simulink model "sampleModel2073"  (R2023a)
settings: Solver=VariableStepAuto  StartTime=0.0  StopTime=10.0  RelTol=1e-3
libraries: hdlsllib x4, simulink x3
settings Model: Creator=user1  LastModifiedBy=user1

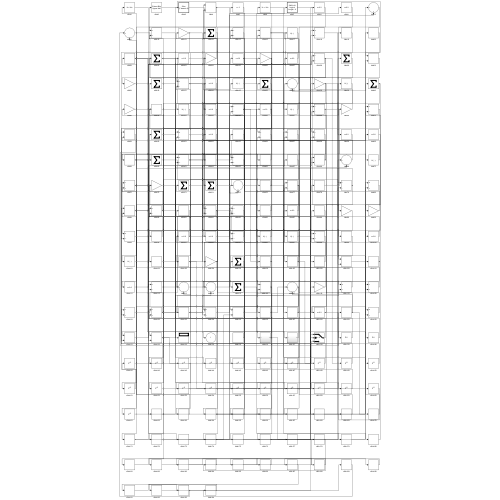
[thumbnail: Simulink's stored preview of the top-level diagram]
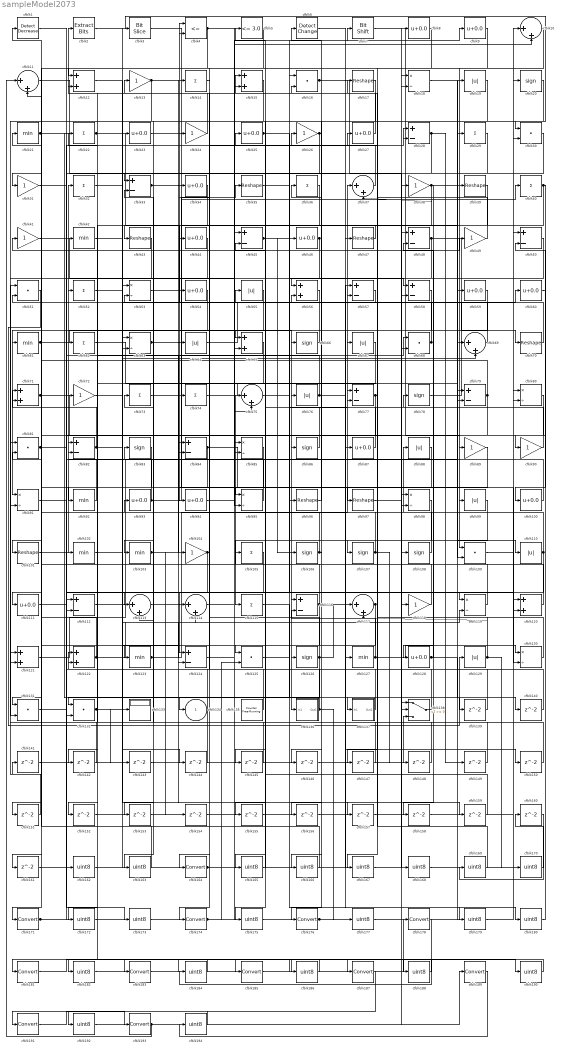
== system sampleModel2073 ==
  cfblk1 : simulink/Logic and Bit Operations/Detect Decrease  vinit=0.0  OutDataTypeStr=boolean
      settings: LibrarySourceBlock=|
      | hdlsllib/Logic and Bit
      | Operations/Detect
      | Decrease
  cfblk{10..11,37,69,75,113..114,117} (8 alike) : Sum  Inputs=|++
  cfblk{8..9,23,25,27,34,44,46,54,59..60,87,93..94,100,111,128} (17 alike) : Bias  Bias=0.0  SaturateOnIntegerOverflow=off
  cfblk{17,35,39,43,47,70,96..97,101} (9 alike) : Reshape
  cfblk{21,42,61,92,102..103,123,127} (8 alike) : MinMax
  cfblk{13,24,26,31,38,41,49,72,89..90,104,118} (12 alike) : Gain
  cfblk{14,22,29,32,36,40,52,62,73..74,105,115} (12 alike) : Sum  Inputs=+
  cfblk{20,66,78,83,86,106..108,126} (9 alike) : Signum
  cfblk{16,30,51,68,81,109,125,131..132} (9 alike) : DotProduct  OutDataTypeStr=Inherit: Inherit via internal rule
  cfblk{19,55,64,67,76,88,99,110,129} (9 alike) : Abs  SaturateOnIntegerOverflow=off
  cfblk{28,33,45,48,50,57..58,77,79,82,84,112,116,124} (14 alike) : Sum  Inputs=+-
  cfblk{18,53,63,80,85,91,95,98,119,130} (10 alike) : Product  Inputs=*/  RndMeth=Zero  SaturateOnIntegerOverflow=on
  cfblk{12,15,56,65,71,120..122} (8 alike) : Sum
  cfblk133 : Display
  cfblk135 : hdlsllib/Sources/Counter Free-Running  NumBits=16  tsamp=-1
  cfblk136 : Subsystem
      settings: LibrarySourceBlock=|
      | hdlsllib/Ports &
      | Subsystems/Subsystem
  cfblk137 : Subsystem
      settings: LibrarySourceBlock=|
      | hdlsllib/Ports &
      | Subsystems/Subsystem
  cfblk138 : Switch  SaturateOnIntegerOverflow=off  InputSameDT=off
  cfblk{139..161} (23 alike) : Delay  SampleTime=1
  cfblk{162..163,165..170,172..173,175,177,179..180,182,184,186,188,190,192,194} (21 alike) : DataTypeConversion  OutDataTypeStr=uint8  SaturateOnIntegerOverflow=off  RndMeth=Floor
  cfblk{164,171,174,176,178,181,183,185,187,189,191,193} (12 alike) : DataTypeConversion  SaturateOnIntegerOverflow=off  RndMeth=Floor
  cfblk2 : simulink/Logic and Bit Operations/Extract Bits  bitsToExtract=Upper half  numBits=8  bitIdxRange=[0 7]  outScalingMode=Preserve fixed-point scaling
      settings: LibrarySourceBlock=|
      | hdlsllib/Logic and Bit
      | Operations/Extract Bits
  cfblk3 : hdlsllib/Logic and Bit Operations/Bit Slice  lidx=7  ridx=0
  cfblk4 : RelationalOperator  Operator=<=  OutDataTypeStr=boolean  InputSameDT=off
  cfblk5 : hdlsllib/Logic and Bit Operations/Compare To Constant  relop=<=  const=3.0  OutDataTypeStr=boolean
  cfblk6 : simulink/Logic and Bit Operations/Detect Change  vinit=0  OutDataTypeStr=boolean
      settings: LibrarySourceBlock=|
      | hdlsllib/Logic and Bit
      | Operations/Detect
      | Change
  cfblk7 : hdlsllib/Logic and Bit Operations/Bit Shift  mode=Shift Left Logical  N=0
  cfblk134 : Outport  VectorParamsAs1DForOutWhenUnconnected=off
  wires:
  cfblk128/1 -> cfblk48/2, cfblk140/1
  cfblk21/1 -> cfblk137/1(In1), cfblk47/1, cfblk84/1
  cfblk93/1 -> cfblk55/1, cfblk12/2
  cfblk111/1 -> cfblk83/1
  cfblk101/1 -> cfblk32/1
  cfblk113/1 -> cfblk37/1
  cfblk10/1 -> cfblk109/1
  cfblk2/1 -> cfblk30/1
  cfblk70/1 -> cfblk4/1
  cfblk47/1 -> cfblk43/1
  cfblk48/1 -> cfblk70/1, cfblk63/2
  cfblk49/1 -> cfblk25/1
  cfblk7/1 -> cfblk89/1
  cfblk108/1 -> cfblk73/1
  cfblk95/1 -> cfblk52/1
  cfblk25/1 -> cfblk125/1, cfblk58/1
  cfblk110/1 -> cfblk88/1, cfblk114/1
  cfblk112/1 -> cfblk18/1
  cfblk59/1 -> cfblk136/1(In1)
  cfblk55/1 -> cfblk91/1
  cfblk16/1 -> cfblk98/1, cfblk119/1
  cfblk120/1 -> cfblk17/1
  cfblk64/1 -> cfblk20/1
  cfblk22/1 -> cfblk94/1, cfblk124/2
  cfblk74/1 -> cfblk76/1
  cfblk53/1 -> cfblk35/1
  cfblk136/1(Out1) -> cfblk34/1, cfblk177/1
  cfblk126/1 -> cfblk13/1, cfblk117/1, cfblk172/1
  cfblk61/1 -> cfblk66/1, cfblk116/1
  cfblk98/1 -> cfblk115/1
  cfblk106/1 -> cfblk21/1, cfblk156/1
  cfblk5/1 -> cfblk164/1
  cfblk78/1 -> cfblk60/1
  cfblk18/1 -> cfblk110/1
  cfblk127/1 -> cfblk130/1, cfblk116/2
  cfblk23/1 -> cfblk86/1
  cfblk51/1 -> cfblk129/1
  cfblk3/1 -> cfblk120/1
  cfblk92/1 -> cfblk82/1
  cfblk24/1 -> cfblk2/1
  cfblk57/1 -> cfblk51/2
  cfblk31/1 -> cfblk24/1
  cfblk11/1 -> cfblk127/1
  cfblk38/1 -> cfblk59/1, cfblk37/2, cfblk84/2, cfblk158/1
  cfblk121/1 -> cfblk29/1
  cfblk102/1 -> cfblk3/1
  cfblk27/1 -> cfblk4/2
  cfblk29/1 -> cfblk112/2
  cfblk71/1 -> cfblk108/1, cfblk173/1
  cfblk54/1 -> cfblk111/1
  cfblk132/1 -> cfblk114/2, cfblk143/1
  cfblk44/1 -> cfblk91/2
  cfblk96/1 -> cfblk6/1
  cfblk28/1 -> cfblk107/1, cfblk134/1, cfblk149/1
  cfblk17/1 -> cfblk113/1
  cfblk116/1 -> cfblk81/2, cfblk145/1, cfblk146/1
  cfblk60/1 -> cfblk100/1
  cfblk37/1 -> cfblk14/1
  cfblk13/1 -> cfblk98/2, cfblk31/1
  cfblk14/1 -> cfblk74/1
  cfblk26/1 -> cfblk33/1, cfblk56/1
  cfblk119/1 -> cfblk75/1
  cfblk40/1 -> cfblk132/1, cfblk90/1
  cfblk88/1 -> cfblk126/1
  cfblk36/1 -> cfblk95/1
  cfblk56/1 -> cfblk113/2
  cfblk39/1 -> cfblk174/1
  cfblk75/1 -> cfblk96/1
  cfblk109/1 -> cfblk130/2
  cfblk82/1 -> cfblk69/2, cfblk71/2
  cfblk138/1 -> cfblk122/1
  cfblk90/1 -> cfblk16/2
  cfblk135/1 -> cfblk93/1
  cfblk89/1 -> cfblk92/1
  cfblk118/1 -> cfblk72/1
  cfblk41/1 -> cfblk75/2
  cfblk130/1 -> cfblk78/1
  cfblk46/1 -> cfblk65/1, cfblk131/2
  cfblk32/1 -> cfblk133/1
  cfblk129/1 -> cfblk26/1, cfblk117/2, cfblk170/1
  cfblk79/1 -> cfblk128/1, cfblk11/2
  cfblk124/1 -> cfblk9/1
  cfblk87/1 -> cfblk41/1
  cfblk137/1(Out1) -> cfblk105/1
  cfblk62/1 -> cfblk109/2
  cfblk63/1 -> cfblk40/1, cfblk95/2
  cfblk123/1 -> cfblk46/1, cfblk119/2
  cfblk125/1 -> cfblk77/1
  cfblk100/1 -> cfblk42/1
  cfblk73/1 -> cfblk104/1
  cfblk34/1 -> cfblk44/1
  cfblk68/1 -> cfblk36/1, cfblk45/2
  cfblk77/1 -> cfblk101/1, cfblk147/1
  cfblk12/1 -> cfblk65/2
  cfblk8/1 -> cfblk61/1
  cfblk91/1 -> cfblk102/1
  cfblk85/1 -> cfblk171/1
  cfblk131/1 -> cfblk27/1
  cfblk107/1 -> cfblk77/2, cfblk148/1
  cfblk19/1 -> cfblk176/1
  cfblk76/1 -> cfblk22/1, cfblk150/1
  cfblk94/1 -> cfblk49/1
  cfblk104/1 -> cfblk54/1, cfblk124/1
  cfblk122/1 -> cfblk57/1, cfblk71/1, cfblk56/2
  cfblk15/1 -> cfblk121/2
  cfblk4/1 -> cfblk97/1, cfblk12/1
  cfblk84/1 -> cfblk103/1, cfblk99/1
  cfblk105/1 -> cfblk132/2
  cfblk69/1 -> cfblk15/1
  cfblk66/1 -> cfblk64/1
  cfblk52/1 -> cfblk28/1
  cfblk86/1 -> cfblk53/2
  cfblk81/1 -> cfblk68/1, cfblk28/2
  cfblk33/1 -> cfblk79/1, cfblk159/1
  cfblk35/1 -> cfblk7/1
  cfblk117/1 -> cfblk123/1, cfblk131/1
  cfblk103/1 -> cfblk67/1, cfblk154/1
  cfblk114/1 -> cfblk10/2
  cfblk45/1 -> cfblk120/2, cfblk106/1
  cfblk115/1 -> cfblk139/1
  cfblk139/1 -> cfblk82/2
  cfblk140/1 -> cfblk112/1
  cfblk141/1 -> cfblk138/2
  cfblk65/1 -> cfblk142/1
  cfblk142/1 -> cfblk51/1
  cfblk42/1 -> cfblk144/1
  cfblk144/1 -> cfblk63/1
  cfblk145/1 -> cfblk53/1
  cfblk146/1 -> cfblk138/3
  cfblk147/1 -> cfblk33/2
  cfblk148/1 -> cfblk122/2
  cfblk149/1 -> cfblk81/1
  cfblk150/1 -> cfblk45/1
  cfblk58/1 -> cfblk151/1
  cfblk151/1 -> cfblk121/1
  cfblk43/1 -> cfblk152/1
  cfblk152/1 -> cfblk16/1
  cfblk67/1 -> cfblk153/1
  cfblk153/1 -> cfblk30/2
  cfblk154/1 -> cfblk68/2
  cfblk99/1 -> cfblk155/1
  cfblk156/1 -> cfblk18/2
  cfblk72/1 -> cfblk157/1
  cfblk157/1 -> cfblk48/1
  cfblk158/1 -> cfblk79/2
  cfblk159/1 -> cfblk15/2
  cfblk83/1 -> cfblk161/1
  cfblk161/1 -> cfblk69/1
  cfblk1/1 -> cfblk162/1
  cfblk162/1 -> cfblk23/1
  cfblk143/1 -> cfblk163/1
  cfblk163/1 -> cfblk1/1
  cfblk164/1 -> cfblk87/1, cfblk138/1
  cfblk30/1 -> cfblk165/1
  cfblk165/1 -> cfblk5/1
  cfblk80/1 -> cfblk166/1
  cfblk166/1 -> cfblk141/1
  cfblk9/1 -> cfblk167/1
  cfblk167/1 -> cfblk80/1
  cfblk97/1 -> cfblk168/1
  cfblk168/1 -> cfblk80/2
  cfblk160/1 -> cfblk169/1
  cfblk169/1 -> cfblk57/2
  cfblk170/1 -> cfblk160/1
  cfblk171/1 -> cfblk62/1, cfblk10/1
  cfblk172/1 -> cfblk85/1
  cfblk173/1 -> cfblk85/2
  cfblk174/1 -> cfblk58/2, cfblk125/2
  cfblk20/1 -> cfblk175/1
  cfblk175/1 -> cfblk39/1
  cfblk176/1 -> cfblk8/1, cfblk118/1
  cfblk177/1 -> cfblk19/1
  cfblk6/1 -> cfblk179/1
  cfblk179/1 -> cfblk50/1
  cfblk155/1 -> cfblk180/1
  cfblk180/1 -> cfblk50/2
  cfblk50/1 -> cfblk182/1
  cfblk182/1 -> cfblk178/1
  cfblk178/1 -> cfblk184/1
  cfblk184/1 -> cfblk181/1
  cfblk181/1 -> cfblk186/1
  cfblk186/1 -> cfblk183/1
  cfblk183/1 -> cfblk188/1
  cfblk188/1 -> cfblk185/1
  cfblk185/1 -> cfblk190/1
  cfblk190/1 -> cfblk187/1
  cfblk191/1 -> cfblk193/1
  cfblk187/1 -> cfblk192/1
  cfblk192/1 -> cfblk189/1
  cfblk193/1 -> cfblk11/1, cfblk38/1
  cfblk189/1 -> cfblk194/1
  cfblk194/1 -> cfblk191/1

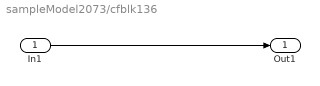
== system sampleModel2073/cfblk136 ==
  In1 : Inport
  Out1 : Outport
  wires:
  In1/1 -> Out1/1

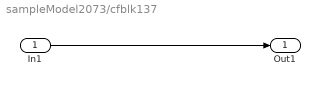
== system sampleModel2073/cfblk137 ==
  In1 : Inport
  Out1 : Outport
  wires:
  In1/1 -> Out1/1
